simulink model "ANC_simulink_5"  (R2023b)
settings: Solver=VariableStepAuto  StartTime=0.0  StopTime=0.5  RelTol=1e-3
values from neighbouring files (symbols this model uses):
  A = 10    [parameter.mat]
  c = 343    [parameter.mat]
  f = 10    [parameter.mat]
  Lp = 1    [parameter.mat]
  Ls = 0.1    [parameter.mat]
  Ts = 0.001    [parameter.mat]
settings Model: Creator=nurbi  LastModifiedBy=nurbi

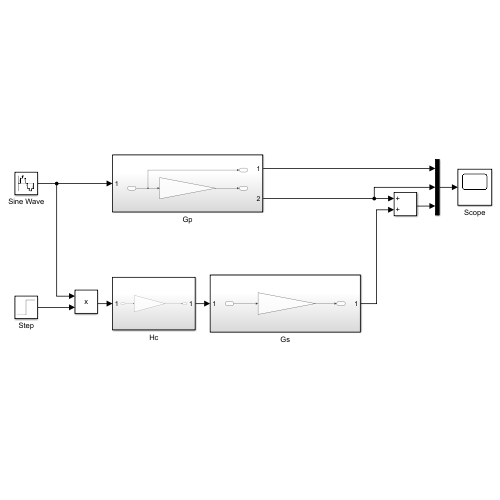
[thumbnail: Simulink's stored preview of the top-level diagram]
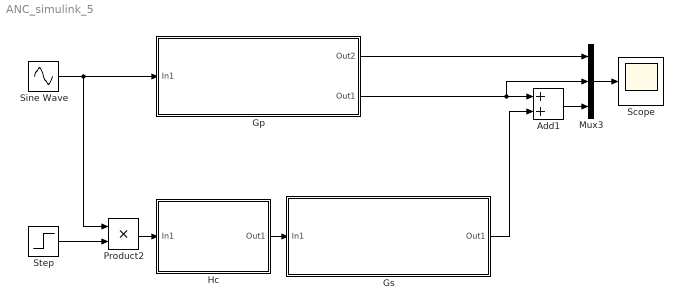
== system ANC_simulink_5 ==
  Add1 : Sum
  Gp : Subsystem
  Gs : Subsystem
  Hc : Subsystem
  Mux3 : Mux  Inputs=3
  Product2 : Product
  Scope : Scope
  Sine Wave : Sin  Amplitude=A  Frequency=2*pi*f  SampleTime=Ts
  Step : Step  Time=0.2  SampleTime=0
  wires:
  Mux3/1 -> Scope/1
  Gp/2(Out1) -> Mux3/2, Add1/1
  Step/1 -> Product2/2
  Hc/1(Out1) -> Gs/1(In1)
  Gs/1(Out1) -> Add1/2
  Sine Wave/1 -> Product2/1, Gp/1(In1)
  Product2/1 -> Hc/1(In1)
  Add1/1 -> Mux3/3
  Gp/1(Out2) -> Mux3/1

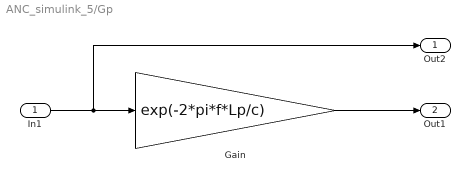
== system ANC_simulink_5/Gp ==
  In1 : Inport
  Gain : Gain  Gain=exp(-2*pi*f*Lp/c)
  Out2 : Outport
  Out1 : Outport  Port=2
  wires:
  In1/1 -> Gain/1, Out2/1
  Gain/1 -> Out1/1

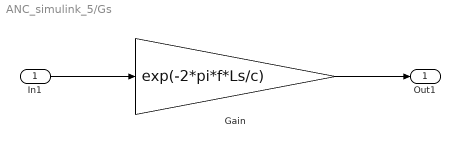
== system ANC_simulink_5/Gs ==
  In1 : Inport
  Gain : Gain  Gain=exp(-2*pi*f*Ls/c)
  Out1 : Outport
  wires:
  In1/1 -> Gain/1
  Gain/1 -> Out1/1

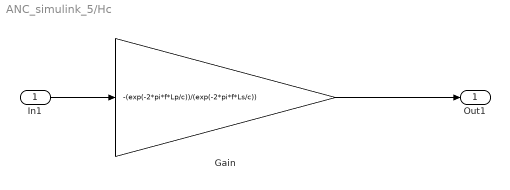
== system ANC_simulink_5/Hc ==
  In1 : Inport
  Gain : Gain  Gain=-(exp(-2*pi*f*Lp/c))/(exp(-2*pi*f*Ls/c))
  Out1 : Outport
  wires:
  Gain/1 -> Out1/1
  In1/1 -> Gain/1
